simulink model "purePursuit"  (R2024b)
settings: Solver=ode4  StartTime=0.0  StopTime=40  FixedStep=1/200  RelTol=1e-3
values from neighbouring files (symbols this model uses):
  a1 = 1    [initialization.m]
  a2 = 2    [initialization.m]
  b1 = 3    [initialization.m]
  b2 = 4    [initialization.m]
  c1 = b1-H    (= 2)    [initialization.m]
  H = 1    [initialization.m]
  l1 = 4    [initialization.m]
  l2 = 6    [initialization.m]
  tau = 0.1    [initialization.m]
settings Model: Creator=sametuslu  LastModifiedBy=sametuslu
settings DataIOCC: ReturnWorkspaceOutputsName=sim

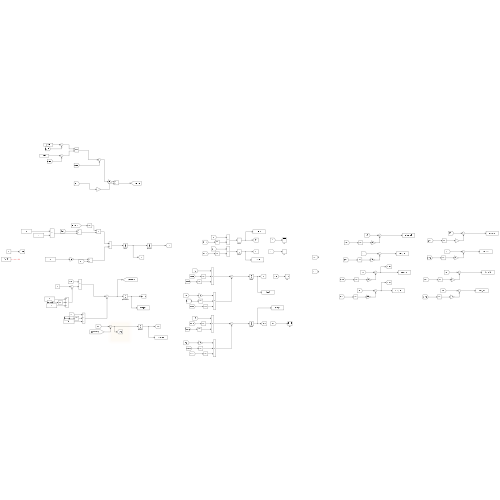
[thumbnail: Simulink's stored preview of the top-level diagram]
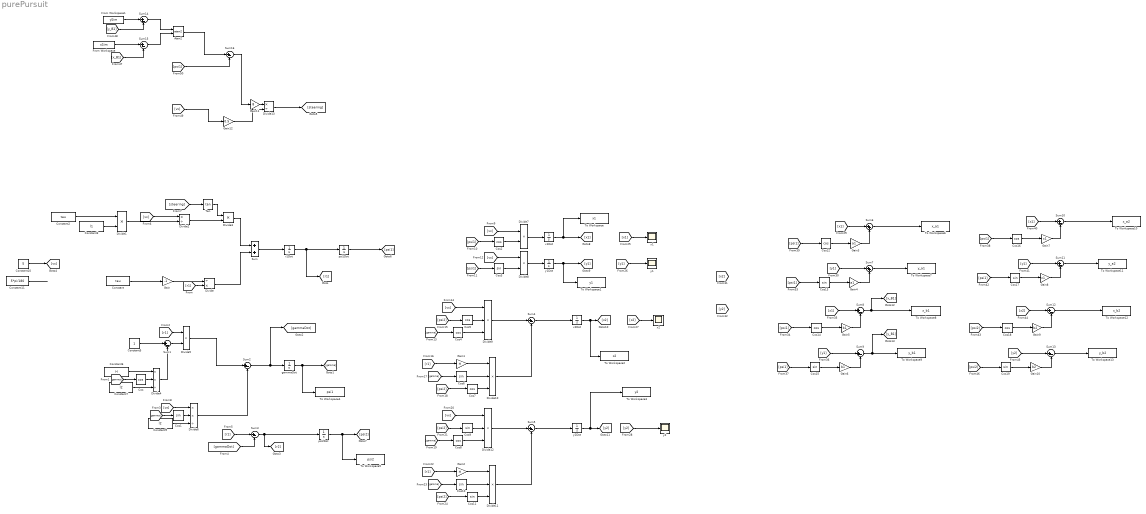
== system purePursuit ==
  Atan2 : Trigonometry  Operator=atan2
  Constant : Constant  Value=tau
  Constant10 : Constant  Value=5
  Constant11 : Constant  Value=5*pi/180
  Constant2 : Constant  Value=tau
  Constant3 : Constant  Value=l1
  Constant5 : Constant
  Constant6 : Constant  Value=H
  Constant7 : Constant  Value=l2
  Constant9 : Constant  Value=l2
  Cos{,2,4..5,7..8,12,14,16,18} (10 alike) : Trigonometry  Operator=cos
  Cos{1,3,6,9..11,13,15,17,19} (10 alike) : Trigonometry
  Divide : Product  Inputs=/*
  Divide{1,3,5,7..8} (5 alike) : Product  Inputs=**
  Divide{9..12} (4 alike) : Product  Inputs=***
  Divide13 : Product  Inputs=*/
  Divide2 : Product  Inputs=*/
  Divide4 : Product  Inputs=**/
  Divide6 : Product  Inputs=**/
  From Workspace : FromWorkspace  VariableName=xSim
  From Workspace1 : FromWorkspace  VariableName=ySim
  Gain : Gain  Gain=-1
  Gain1 : Gain  Gain=H
  Gain10 : Gain  Gain=b2
  Gain11 : Gain  Gain=8
  Gain12 : Gain  Gain=0.5
  Gain2 : Gain  Gain=H
  Gain3 : Gain  Gain=a1
  Gain4 : Gain  Gain=a1
  Gain5 : Gain  Gain=b1
  Gain6 : Gain  Gain=b1
  Gain7 : Gain  Gain=c1
  Gain8 : Gain  Gain=c1
  Gain9 : Gain  Gain=b2
  Sum : Sum
  Sum{1..5,8..16} (14 alike) : Sum  Inputs=|+-
  Sum6 : Sum  Inputs=|++
  Sum7 : Sum  Inputs=|++
  Tan : Trigonometry  Operator=tan
  To Workspace : ToWorkspace  VariableName=x1  SampleTime=-1
  To Workspace1 : ToWorkspace  VariableName=y1  SampleTime=-1
  To Workspace10 : ToWorkspace  VariableName=x_a2  SampleTime=-1
  To Workspace11 : ToWorkspace  VariableName=y_a2  SampleTime=-1
  To Workspace12 : ToWorkspace  VariableName=x_b2  SampleTime=-1
  To Workspace13 : ToWorkspace  VariableName=y_b2  SampleTime=-1
  To Workspace2 : ToWorkspace  VariableName=x2  SampleTime=-1
  To Workspace3 : ToWorkspace  VariableName=y2  SampleTime=-1
  To Workspace4 : ToWorkspace  VariableName=psi1  SaveFormat=Timeseries  SampleTime=-1
  To Workspace5 : ToWorkspace  VariableName=psi2  SaveFormat=Timeseries  SampleTime=-1
  To Workspace6 : ToWorkspace  VariableName=x_a1  SampleTime=-1
  To Workspace7 : ToWorkspace  VariableName=y_a1  SampleTime=-1
  To Workspace8 : ToWorkspace  VariableName=x_b1  SampleTime=-1
  To Workspace9 : ToWorkspace  VariableName=y_b1  SampleTime=-1
  gammaDot : Integrator
  psi1Dot : Integrator
  psi2Dot : Integrator
  r1Dot : Integrator
  x1 : Scope
  x1Dot : Integrator
  x2 : Scope
  x2Dot : Integrator  InitialCondition=-c1-a2
  y1 : Scope
  y1Dot : Integrator
  y2 : Scope
  y2Dot : Integrator
  wires:
  Sum/1 -> r1Dot/1
  r1Dot/1 -> psi1Dot/1, [r1]
  Constant/1 -> Gain/1
  Gain/1 -> Divide/1
  Constant2/1 -> Divide1/1
  Constant3/1 -> Divide1/2
  [vx] -> Divide2/1
  Divide1/1 -> Divide2/2
  Divide2/1 -> Divide3/2
  [steering] -> Tan/1
  Tan/1 -> Divide3/1
  Divide3/1 -> Sum/1
  Divide/1 -> Sum/2
  Constant5/1 -> Sum1/1
  Constant6/1 -> Divide4/1
  Cos/1 -> Divide4/2
  [r1] -> Divide/2
  gammaDot/1 -> To Workspace4/1, [gamma]
  [gamma] -> Cos/1
  Constant7/1 -> Divide4/3
  Divide4/1 -> Sum1/2
  [r1] -> Divide5/1
  Sum1/1 -> Divide5/2
  [vx] -> Divide6/1
  Constant9/1 -> Divide6/3
  Cos1/1 -> Divide6/2
  [gamma] -> Cos1/1
  Sum2/1 -> [gammaDot], gammaDot/1
  Divide5/1 -> Sum2/1
  Divide6/1 -> Sum2/2
  [r1] -> Sum3/1
  [gammaDot] -> Sum3/2
  Sum3/1 -> [r2], psi2Dot/1
  Constant10/1 -> [vx]
  Constant11/1 -> ?
  psi1Dot/1 -> [psi1]
  psi2Dot/1 -> To Workspace5/1, [psi2]
  [psi1] -> Cos2/1
  Cos2/1 -> Divide7/2
  [vx] -> Divide7/1
  Divide7/1 -> x1Dot/1
  x1Dot/1 -> To Workspace/1, [x1]
  Divide8/1 -> y1Dot/1
  [vx] -> Divide8/1
  Cos3/1 -> Divide8/2
  [psi1] -> Cos3/1
  y1Dot/1 -> To Workspace1/1, [y1]
  [gamma] -> Cos4/1
  Cos4/1 -> Divide9/3
  [vx] -> Divide9/1
  [psi2] -> Cos5/1
  Cos5/1 -> Divide9/2
  Divide9/1 -> Sum4/1
  [r1] -> Gain1/1
  Gain1/1 -> Divide10/1
  [gamma] -> Cos6/1
  Cos6/1 -> Divide10/2
  [psi2] -> Cos7/1
  Cos7/1 -> Divide10/3
  Divide10/1 -> Sum4/2
  Sum4/1 -> x2Dot/1
  Sum5/1 -> y2Dot/1
  Divide11/1 -> Sum5/2
  Cos11/1 -> Divide11/3
  [psi2] -> Cos11/1
  Cos10/1 -> Divide11/2
  [gamma] -> Cos10/1
  Gain2/1 -> Divide11/1
  [r1] -> Gain2/1
  Divide12/1 -> Sum5/1
  Cos9/1 -> Divide12/2
  [psi2] -> Cos9/1
  [vx] -> Divide12/1
  Cos8/1 -> Divide12/3
  [gamma] -> Cos8/1
  x2Dot/1 -> To Workspace2/1, [x2]
  y2Dot/1 -> To Workspace3/1, [y2]
  [x1] -> x1/1
  [y1] -> y1/1
  [x2] -> x2/1
  [y2] -> y2/1
  [x1] -> Sum6/1
  [psi1] -> Cos12/1
  Cos12/1 -> Gain3/1
  Gain3/1 -> Sum6/2
  Sum6/1 -> To Workspace6/1
  [y1] -> Sum7/1
  Cos13/1 -> Gain4/1
  [psi1] -> Cos13/1
  Gain4/1 -> Sum7/2
  Sum7/1 -> To Workspace7/1
  Sum9/1 -> [y_B1], To Workspace9/1
  Gain6/1 -> Sum9/2
  [psi1] -> Cos15/1
  Cos15/1 -> Gain6/1
  [y1] -> Sum9/1
  Sum8/1 -> [x_B1], To Workspace8/1
  Gain5/1 -> Sum8/2
  Cos14/1 -> Gain5/1
  [psi1] -> Cos14/1
  [x1] -> Sum8/1
  [x1] -> Sum10/1
  [psi1] -> Cos16/1
  Cos16/1 -> Gain7/1
  Gain7/1 -> Sum10/2
  Sum10/1 -> To Workspace10/1
  [y1] -> Sum11/1
  Cos17/1 -> Gain8/1
  [psi1] -> Cos17/1
  Gain8/1 -> Sum11/2
  Sum11/1 -> To Workspace11/1
  [x2] -> Sum12/1
  [psi2] -> Cos18/1
  Cos18/1 -> Gain9/1
  Gain9/1 -> Sum12/2
  Sum12/1 -> To Workspace12/1
  [y2] -> Sum13/1
  Cos19/1 -> Gain10/1
  [psi2] -> Cos19/1
  Gain10/1 -> Sum13/2
  Sum13/1 -> To Workspace13/1
  From Workspace1/1 -> Sum14/1
  [y_B1] -> Sum14/2
  Sum14/1 -> Atan2/1
  From Workspace/1 -> Sum15/1
  [x_B1] -> Sum15/2
  Sum15/1 -> Atan2/2
  Atan2/1 -> Sum16/1
  Gain11/1 -> Divide13/1
  [vx] -> Gain12/1
  Divide13/1 -> [steering]
  [psi1] -> Sum16/2
  Sum16/1 -> Gain11/1
  Gain12/1 -> Divide13/2
